simulink model "StateSpaceRepDCMotor"  (R2021a)
settings: Solver=VariableStepAuto  StartTime=0.0  StopTime=10.0  RelTol=1e-3
values from neighbouring files (symbols this model uses):
  A = [0      1       0 ... (first row only)    [StateSpaceRepresentation.m]
  B = [  0      1 ... (first row only)    [StateSpaceRepresentation.m]
  C = [ 0 1 0 ... (first row only)    [StateSpaceRepresentation.m]
  D = [ 0 0 ... (first row only)    [StateSpaceRepresentation.m]
undefined symbols (not defined in the file or in its folder): den, num
settings Model: Creator=HP  LastModifiedBy=HP

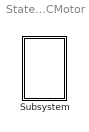
== system StateSpaceRepDCMotor ==
  Subsystem : Subsystem

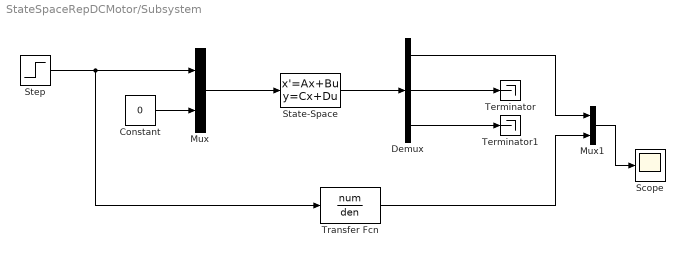
== system StateSpaceRepDCMotor/Subsystem ==
  Constant : Constant  Value=0
  Demux : Demux  Outputs=3
  Mux : Mux  Inputs=2
  Mux1 : Mux  Inputs=2
  Scope : Scope
  State-Space : StateSpace  A=A  B=B  C=C  D=D  InitialCondition=0
  Step : Step  SampleTime=0
  Terminator : Terminator
  Terminator1 : Terminator
  Transfer Fcn : TransferFcn  Numerator=num  Denominator=den
  wires:
  Demux/3 -> Terminator1/1
  Step/1 -> Transfer Fcn/1, Mux/1
  Demux/1 -> Mux1/1
  Constant/1 -> Mux/2
  Mux1/1 -> Scope/1
  Demux/2 -> Terminator/1
  State-Space/1 -> Demux/1
  Mux/1 -> State-Space/1
  Transfer Fcn/1 -> Mux1/2
